simulink model "Model_Tracking"  (R2022b)
settings: Solver=VariableStepAuto  StartTime=0.0  StopTime=10.0  RelTol=1e-3
values from neighbouring files (symbols this model uses):
  X0 = [10; 0; 0; 0; 1000]    [Controladores.m]    (also in UAV.m)
undefined symbols (not defined in the file or in its folder): A, B, C, D
settings Model: Creator=samue  LastModifiedBy=samue

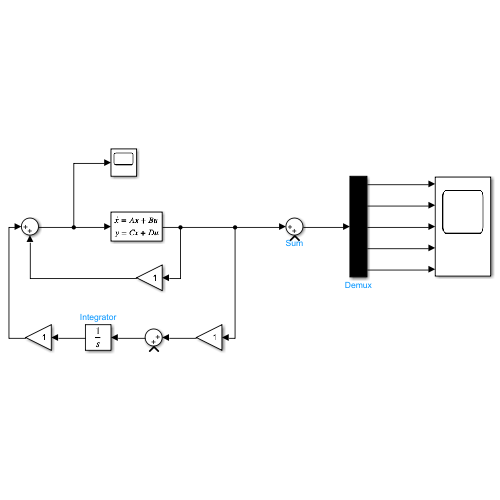
[thumbnail: Simulink's stored preview of the top-level diagram]
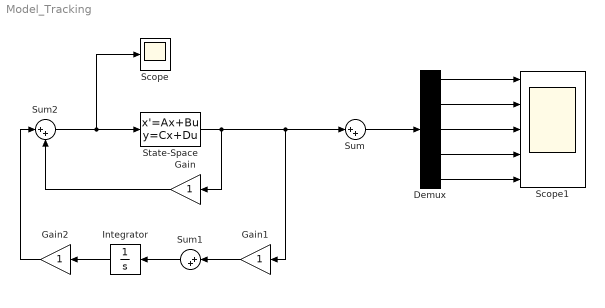
== system Model_Tracking ==
  Demux : Demux  Outputs=5
  Gain : Gain
  Gain1 : Gain
  Gain2 : Gain
  Integrator : Integrator
  Scope : Scope
  Scope1 : Scope  NumInputPorts=5
  State-Space : StateSpace  A=A  B=B  C=C  D=D  InitialCondition=X0  ParameterTunability=Unconstrained
  Sum : Sum  Inputs=|++
  Sum1 : Sum  Inputs=|++
  Sum2 : Sum  Inputs=|++
  wires:
  Sum/1 -> Demux/1
  State-Space/1 -> Gain/1, Gain1/1, Sum/1
  Sum2/1 -> State-Space/1, Scope/1
  Gain2/1 -> Sum2/1
  Gain/1 -> Sum2/2
  Integrator/1 -> Gain2/1
  Sum1/1 -> Integrator/1
  Gain1/1 -> Sum1/1
  Demux/1 -> Scope1/1
  Demux/2 -> Scope1/2
  Demux/3 -> Scope1/3
  Demux/4 -> Scope1/4
  Demux/5 -> Scope1/5
